simulink model "Feeder_1"  (Simulink 8.8)
settings: Solver=ode4  StartTime=0.0  StopTime=inf  FixedStep=Ts  RelTol=1e-3  EnableMultiTasking=on
PreLoadFcn:
  | Ts=125e-6;Core_Num = 0; np=1; nq=1; Vmin=.9;
PostLoadFcn:
  | Ts=125e-6;Core_Num = 0; np=1; nq=1; Vmin=.9;
InitFcn:
  | Ts=125e-6;Core_Num = 0; np=1; nq=1; Vmin=.9;
undefined symbols (not defined in the file or in its folder): another_event_name, DiscIntNeverNeededParam, I, j, Left, my_event_name, Right, type, V, X
libraries: powerlib x316, powerlib_meascontrol x227, simulink_extras x78, simulink x25, rtio_generic_c37_118 x22, ssn_lib x9, rtlab x6, powerlib_extras x3, artemis x1, rtio_opalrt_ml605ex1 x1, rtio_spectracom x1, rtio_generic_ethernet x1
(part 1 of 14)
settings Model: ARTEMISmethode_block_infos=$$__separator__$$Feeder_1/ARTEMIS Guide1$$__separator__$$  Creator=DETLDAQ  LastModifiedBy=rdarbal
settings OptimizationCC: BlockReduction=off  BooleanDataType=off  OptimizeBlockIOStorage=off  BufferReuse=off  GlobalBufferReuse=off  ExpressionFolding=off  LocalBlockOutputs=off
settings DebuggingCC: SaveWithParameterizedLinksMsg=none  SignalResolutionControl=TryResolveAllWithWarning  MultiTaskDSMMsg=warning  MultiTaskCondExecSysMsg=none  FcnCallInpInsideContextMsg=error
settings HardwareCC: TargetBitPerPointer=64  TargetBitPerSizeT=64  TargetBitPerPtrDiffT=64  TargetLongLongMode=on  TargetIntDivRoundTo=Zero  TargetEndianess=LittleEndian  TargetWordSize=64  TargetHWDeviceType=MATLAB Host  ProdEqTarget=off
settings GRTTargetCC: CombineOutputUpdateFcns=on  GRTInterface=off

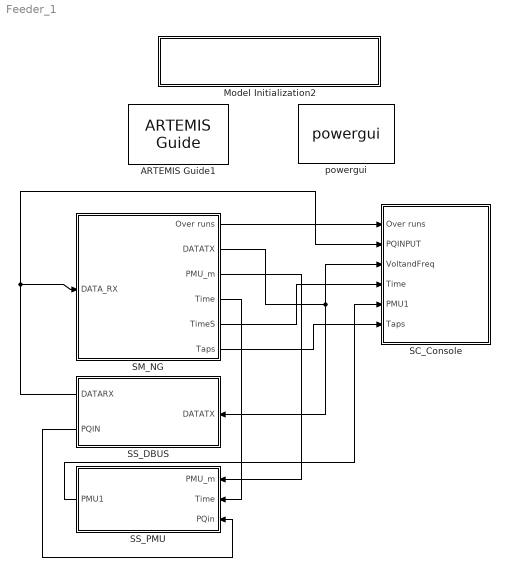
== system Feeder_1 ==
  ARTEMIS Guide1 : artemis/ARTEMIS/ARTEMIS Guide  Tag=FTSSmethode_opal_4hx0r99  Description=5.0_z1  lock=on  Ts=Ts  opt=art5  dyna=off  nb_perm=4  RT_fullcomp=off  ssn=on  ssn_itvc=off  ssn_ivic=off  ssn_ext=off  ssn_solver=Backward Euler  ssn_impulse=off  ssn_quasimpulse=off  ssn_impulse_loop=5  paraExtinctionThy=off  Thy_Impulse=off  dtc=Off  dtc_opt=normal  ao=on  simtype=off  ct_mac=off  lin_mov=off  lsp=[0.001 2]  spike_skip=Disabled  dtc_extra=1  dtc_sws=normal  dtc_pied=0.5  SPSRulesBlock=SPSRules  tre=off  ctmm=off  LF=on  dpl_type=ARTEMiS DPL  rlc_type=off  custom_type=off  para=on  ssn_ImpulseLoopBlockedStateUpdate=5  ssn_mov_iter_number=5  ssn_switch_iter_number=5  ssn_nib_type_verify=on  ssn_use_lu=on  ssn_use_ldlt=off
  Model Initialization2 : Subsystem  AncestorBlock=artemis/Tools /Misc/Model Initialization  mask(Model Functions){InitFcnX=Ts=125e-6;Core_Num = 0; np=1; nq=1; Vmin=.9;, prel=on, posl=on, inif=on, strf=off}
      mask prompts: InitFcnX "Initialisation"; prel "Preload Function"; posl "PostLoad Function"; inif "InitFcn"; strf "StartFcn"
      mask init:
      | currentBlock = gcb;
      | root = bdroot(currentBlock);
      | 
      | if ~strcmp(get_param(root,'BlockDiagramType'),'library')
      |     if prel==1
      |         set_param(root, 'PreLoadFcn', InitFcnX);
      |     else
      |         set_param(root, 'PreLoadFcn', '');
      |     end
      |     if inif==1
      |         set_param(root, 'InitFcn', InitFcnX);
      |     else
      |         set_param(root, 'InitFcn', '');
      |     end
      |     if strf==1
      |         set_param(root, 'StartFcn', InitFcnX);
      |     else
      |         set_param(root, 'StartFcn', '');
      |     end
      |     if posl==1
      |         set_param(root, 'PostLoadFcn', InitFcnX);
      |     else
      |         set_param(root, 'PostLoadFcn', '');
      |     end
      | end
      | 
      | pos = get_param(currentBlock, 'Position');
      | width = pos(3) - pos(1); height = pos(4) - pos(2);
      | txt = [ upper(root) '\n' '- InitFcn. . . . . '  get_param(root, 'InitFcn') ];
      settings: CopyFcn=set_param(gcb,'LinkStatus','inactive')
      mask Display: text(5, height*0.5, txt, 'horizontalAlignment', 'left', 'verticalAlignment', 'middle') ;
  SC_Console : Subsystem
  SM_NG : Subsystem
  SS_DBUS : Subsystem
  SS_PMU : Subsystem
  powergui : powerlib/powergui  Priority=1  SimulationMode=Discrete  SolverType=Backward Euler  SampleTime=Ts  frequency=60  SPID=off  DisableSnubberDevices=off  DisableRonSwitches=off  DisableVfSwitches=off  SwTol=0  DisplayEquations=off  Interpol=off  ExternalGateDelay=off  methode=off  Ts=100  FunctionMessages=off  echomessages=off  HookPort=off  EnableUseOfTLC=off  x0status=blocks  frequencyindice=0  Pbase=100e6  ErrMax=1e-4  Iterations=50  UnitsV=kV  UnitsW=MW  buscounter=0  RestoreLinks=warning  ResistiveCurrentMeasurement=off  Frange=[0:2:500]  Ylog=off  Xlog=on  ShowGrid=off  save=off  variable=ZData  structure=0  ZoomFFT=off  StartTime=0.0  cycles=1  DisplayStyle=1  fundamental=60  FreqAxis=off  MaxFrequency=1000  frequencyindicesteady=1  RmsSteady=1  display=off
  wires:
  SS_DBUS/1(DATARX) -> SC_Console/2(PQINPUT), SM_NG/1(DATA_RX)
  SM_NG/2(DATATX) -> SS_DBUS/1(DATATX), SC_Console/3(VoltandFreq)
  SM_NG/3("PMU_m ") -> SS_PMU/1(PMU_m)
  SM_NG/4(Time) -> SS_PMU/2(Time)
  SM_NG/1(Over runs) -> SC_Console/1(Over runs)
  SM_NG/5(TimeS) -> SC_Console/4(Time)
  SS_PMU/1(PMU1) -> SC_Console/5(PMU1)
  SS_DBUS/2(PQIN) -> SS_PMU/3(PQin)
  SM_NG/6(Taps) -> SC_Console/6(Taps)

== system Feeder_1/Model Initialization2 ==

== system Feeder_1/SC_Console ==
  Over runs : Inport
  PQINPUT : Inport  Port=2
  VoltandFreq : Inport  Port=3
  Time : Inport  Port=4
  PMU1 : Inport  Port=5
  Taps : Inport  Port=6
  Demux2 : Demux  Outputs=8
  Display{,1..3,15..22} (12 alike) : Display
  OpComm1 : rtlab/OpComm  nbport=6  groupe_acq=1  subsys_rate=0  st=0  Synchronization=on  Interpolation=on  Threshold=1.0  Missed_Data=off  Sim_Time=off  Samples=off  dynSigOut=off  from_console=0  warning_done=off  writeOpCommFile=off  Offset=off
  "Tap " : Display
  wires:
  Over runs/1 -> OpComm1/1
  PQINPUT/1 -> OpComm1/2
  OpComm1/1 -> Display/1
  OpComm1/2 -> Display1/1
  VoltandFreq/1 -> OpComm1/3
  OpComm1/3 -> Display2/1
  Time/1 -> OpComm1/4
  OpComm1/4 -> [TimeStamp]
  [TimeStamp] -> Demux2/1
  Demux2/1 -> Display15/1
  Demux2/2 -> Display16/1
  Demux2/3 -> Display17/1
  Demux2/4 -> Display18/1
  Demux2/5 -> Display19/1
  Demux2/6 -> Display20/1
  Demux2/7 -> Display21/1
  Demux2/8 -> Display22/1
  PMU1/1 -> OpComm1/5
  OpComm1/5 -> Display3/1
  Taps/1 -> OpComm1/6
  OpComm1/6 -> "Tap "/1
